simulink model "RCAM_simulation"  (R2021b)
settings: Solver=VariableStepAuto  StartTime=0.0  StopTime=TF  RelTol=1e-3
values from neighbouring files (symbols this model uses):
  h0 = 0    [initializeConstants.m]
  lat0 = convert_coordinates(21, 18, 56.1708)    [initializeConstants.m]
  lon0 = convert_coordinates(157, 51, 29.1348)    [initializeConstants.m]
  u1max = 25*pi/180    (= 0.436332312999)    [initializeConstants.m]
  u1min = -25*pi/180    (= -0.436332312999)    [initializeConstants.m]
  u2max = 10*pi/180    (= 0.174532925199)    [initializeConstants.m]
  u2min = -25*pi/180    (= -0.436332312999)    [initializeConstants.m]
  u3max = 30*pi/180    (= 0.523598775598)    [initializeConstants.m]
  u3min = -30*pi/180    (= -0.523598775598)    [initializeConstants.m]
  u4max = 10*pi/180    (= 0.174532925199)    [initializeConstants.m]
  u4min = 0    [initializeConstants.m]
  u5max = 10*pi/180    (= 0.174532925199)    [initializeConstants.m]
  u5min = 0    [initializeConstants.m]
  udist = [10 ... (first row only)    [initializeConstants.m]
  uo = [0; -0.1780; 0; 0.0821; 0.0821]    [initializeConstants.m]
  x0 = [84.9905; 0; 1.2713; 0; 0; 0; 0; 0.0150; 0]    [initializeConstants.m]
undefined symbols (not defined in the file or in its folder): RCAM_model
libraries: aerolibfltsims x2
settings Model: Creator=khanh  LastModifiedBy=khanh

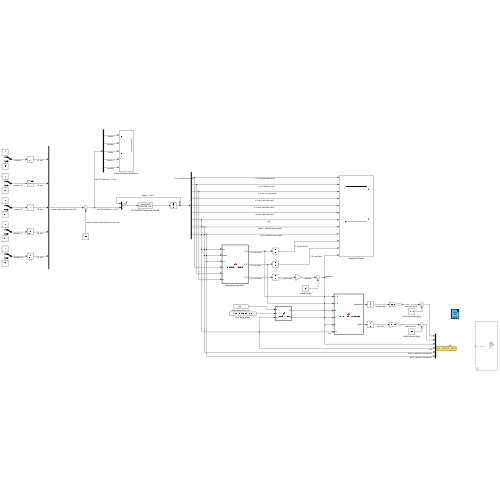
[thumbnail: Simulink's stored preview of the top-level diagram]
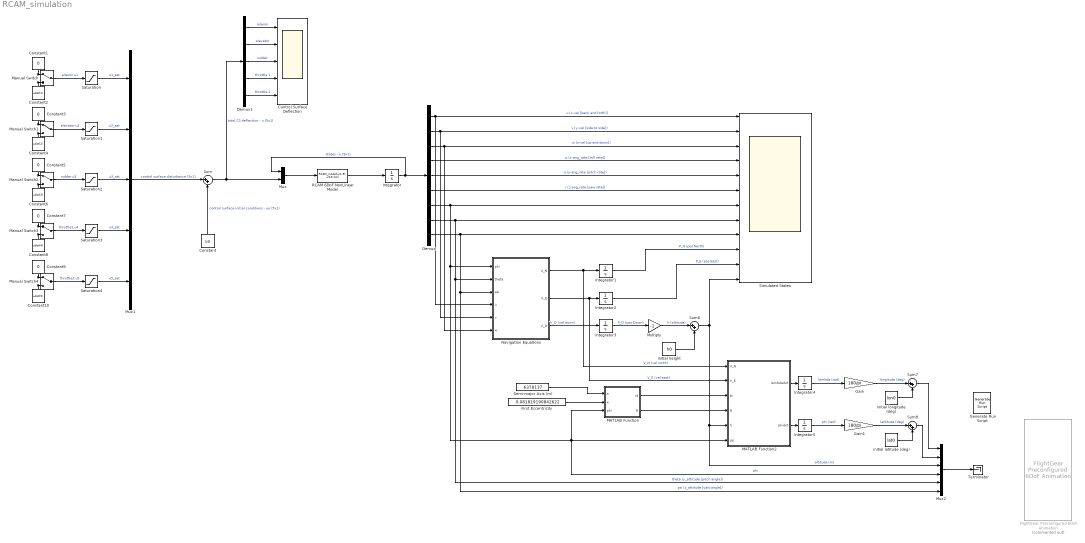
== system RCAM_simulation ==
  Constant : Constant  Value=uo
  Constant{1,3,5,7,9} (5 alike) : Constant  Value=0
  Constant10 : Constant  Value=udist(5)
  Constant2 : Constant  Value=udist(1)
  Constant4 : Constant  Value=udist(2)
  Constant6 : Constant  Value=udist(3)
  Constant8 : Constant  Value=udist(4)
  Control Surface Deflection : Scope  NumInputPorts=5
  Demux : Demux  Outputs=9
  Demux1 : Demux  Outputs=5
  First Eccentricity : Constant  Value=0.081819190842622
  FlightGear Preconfigured 6DoF Animation : aerolibfltsims/FlightGear Preconfigured 6DoF Animation  Commented=on  xFlightGearVersion=v2019.1  DestinationIpAddress=127.0.0.1  DestinationPort=5502  SampleTime=1/30  packetVersion=24
  Gain : Gain  Gain=180/pi
  Gain1 : Gain  Gain=180/pi
  Generate Run Script : aerolibfltsims/Generate Run Script  Architecture=Win64  dataFlow=Send  GeometryModelName=c172p  AirportId=KSFO  RunwayId=10L  InitialAltitude=7224  InitialHeading=113  OffsetDistance=4.72  OffsetAzimuth=0  InstallScenery=off  DisableShaders=on  OriginAddress=127.0.0.1  DestinationPort=5502  OriginPort=5505  LocalAddress=127.0.0.1  OutputFileName=runfg.bat  FlightGearBaseDirectory=C:\Program Files\FlightGear 2020.3
  Integrator : Integrator  InitialCondition=x0
  Integrator{1..4} (4 alike) : Integrator
  Integrator5 : Integrator  UpperSaturationLimit=pi  LowerSaturationLimit=-pi
  MATLAB Function : MATLAB Function  TreatAsAtomicUnit=on
  MATLAB Function2 : MATLAB Function  TreatAsAtomicUnit=on
  Manual Switch{,1..4} (5 alike) : ManualSwitch
  Multiply : Gain  Gain=-1
  Mux : Mux  Inputs=2
  Mux1 : Mux  Inputs=5
  Mux2 : Mux  Inputs=6
  Navigation Equations : MATLAB Function  TreatAsAtomicUnit=on
  RCAM 6DoF NonLinear Model : MATLABFcn  MATLABFcn=RCAM_model(u(1:9), u(10:14))
  Saturation : Saturate  UpperLimit=u1max  LowerLimit=u1min
  Saturation1 : Saturate  UpperLimit=u2max  LowerLimit=u2min
  Saturation2 : Saturate  UpperLimit=u3max  LowerLimit=u3min
  Saturation3 : Saturate  UpperLimit=u4max  LowerLimit=u4min
  Saturation4 : Saturate  UpperLimit=u5max  LowerLimit=u5min
  Semi-major Axis (m) : Constant  Value=6378137
  Simulated States : Scope  NumInputPorts=12
  Sum{,6..8} (4 alike) : Sum  Inputs=|++
  Terminator : Terminator
  initial height : Constant  Value=h0
  initial latitude (deg) : Constant  Value=lat0
  initial longitude (deg) : Constant  Value=lon0
  wires:
  RCAM 6DoF NonLinear Model/1 -> Integrator/1
  Integrator/1 -> Demux/1, Mux/1  "states - x (9x1)"
  Constant/1 -> Sum/2  "control surface initial conditions - uo (5x1)"
  Mux/1 -> RCAM 6DoF NonLinear Model/1
  Sum/1 -> Demux1/1, Mux/2  "total CS deflection - u (5x1)"
  Constant2/1 -> Manual Switch/2
  Constant1/1 -> Manual Switch/1
  Manual Switch/1 -> Saturation/1  "aileron u1"
  Saturation/1 -> Mux1/1  "u1_sat"
  Manual Switch4/1 -> Saturation4/1  "throttle2 u5"
  Saturation4/1 -> Mux1/5  "u5_sat"
  Saturation3/1 -> Mux1/4  "u4_sat"
  Manual Switch3/1 -> Saturation3/1  "throttle1 u4"
  Manual Switch2/1 -> Saturation2/1  "rudder u3"
  Saturation2/1 -> Mux1/3  "u3_sat"
  Saturation1/1 -> Mux1/2  "u2_sat"
  Demux1/1 -> Control Surface Deflection/1  "aileron"
  Demux1/2 -> Control Surface Deflection/2  "elevator"
  Demux1/3 -> Control Surface Deflection/3  "rudder"
  Demux1/4 -> Control Surface Deflection/4  "throttle 1"
  Demux1/5 -> Control Surface Deflection/5  "throttle 2"
  Mux1/1 -> Sum/1  "control surface disturbance (5x1)"
  Demux/1 -> Navigation Equations/4(u), Simulated States/1  "u (x-vel [back and forth])"
  Demux/2 -> Navigation Equations/5(v), Simulated States/2  "v (y-vel [side to side])"
  Demux/3 -> Navigation Equations/6(w), Simulated States/3  "w (z-vel [up and down])"
  Demux/4 -> Simulated States/4  "p (x-ang_rate [roll rate])"
  Demux/5 -> Simulated States/5  "q (y-ang_rate [pitch rate])"
  Demux/6 -> Simulated States/6  "r (z-ang_rate [yaw rate])"
  Demux/8 -> Mux2/5, Navigation Equations/2(theta), Simulated States/8  "theta (y_attitude [pitch angle])"
  Demux/9 -> Mux2/6, Navigation Equations/3(psi), Simulated States/9  "psi (z_attitude [yaw angle])"
  Navigation Equations/3(V_D) -> Integrator3/1  "V_D (vel down)"
  Navigation Equations/2(V_E) -> Integrator2/1, MATLAB Function2/2(V_E)  "V_E (vel east)"
  Navigation Equations/1(V_N) -> MATLAB Function2/1(V_N), Integrator1/1  "V_N (vel north)"
  Integrator1/1 -> Simulated States/10  "P_N (pos North)"
  Integrator2/1 -> Simulated States/11  "P_E (pos East)"
  Integrator3/1 -> Multiply/1  "P_D (pos Down)"
  Semi-major Axis (m)/1 -> MATLAB Function/1(a)
  First Eccentricity/1 -> MATLAB Function/2(e)
  MATLAB Function/2(N) -> MATLAB Function2/4(N)
  MATLAB Function/1(M) -> MATLAB Function2/3(M)
  Demux/7 -> MATLAB Function2/6(psi), MATLAB Function/3(phi), Mux2/4, Navigation Equations/1(phi), Simulated States/7  "phi"
  Integrator5/1 -> Gain1/1  "phi (rad)"
  Integrator4/1 -> Gain/1  "lambda (rad)"
  Gain/1 -> Sum7/1  "longitude (deg)"
  Multiply/1 -> Sum6/1  "h (altitude)"
  Sum6/1 -> Simulated States/12, Mux2/3, MATLAB Function2/5(h)  "altitude (m)"
  initial height/1 -> Sum6/2
  MATLAB Function2/1(lambdadot) -> Integrator4/1
  MATLAB Function2/2(phidot) -> Integrator5/1
  Gain1/1 -> Sum8/1  "lattitude (deg)"
  initial longitude (deg)/1 -> Sum7/2
  initial latitude (deg)/1 -> Sum8/2
  Sum7/1 -> Mux2/1
  Sum8/1 -> Mux2/2
  Constant4/1 -> Manual Switch1/2
  Constant3/1 -> Manual Switch1/1
  Constant6/1 -> Manual Switch2/2
  Constant5/1 -> Manual Switch2/1
  Constant8/1 -> Manual Switch3/2
  Constant7/1 -> Manual Switch3/1
  Constant10/1 -> Manual Switch4/2
  Constant9/1 -> Manual Switch4/1
  Manual Switch1/1 -> Saturation1/1  "elevator u2"
  Mux2/1 -> Terminator/1

== matlab function RCAM_simulation/MATLAB Function ==
  data: a input; M output; e input; phi input; N output
function [M, N] = calculate_mn (a, e, phi)

M = a*(1-e^2)/(1-(e^2)*sin(phi)^2)^1.5;

N = a/(1-(e^2)*sin(phi)^2)^0.5;

end

== matlab function RCAM_simulation/Navigation Equations ==
  data: phi input; theta input; psi input; u input; V_N output; v input; w input; V_E output; V_D output
function [V_N, V_E, V_D] = navigation_equation(phi, theta, psi, u, v, w)

x7 = phi;
x8 = theta;
x9 = psi;
x1 = u;
x2 = v;
x3 = w;

V_b = [x1; x2; x3];

%navigation equations
C1v = [cos(x9) sin(x9) 0; -sin(x9) cos(x9) 0; 0 0 1];

C21 = [cos(x8) 0 -sin(x8); 0 1 0; sin(x8) 0 cos(x8)];

Cb2 = [1 0 0; 0 cos(x7) sin(x7); 0 -sin(x7) cos(x7)];

Cvb = Cb2*C21*C1v;
Cvb = Cvb';

vel_vector = Cvb*V_b;

V_N = vel_vector(1);
V_E = vel_vector(2);
V_D = vel_vector(3);

end

== matlab function RCAM_simulation/MATLAB Function2 ==
  data: lambdadot output; V_N input; V_E input; phidot output; M input; N input; h input; psi input
function [lambdadot, phidot] = calculate_phi_lambdadot(V_N, V_E, M, N, h, psi)

lambdadot = V_E/(N+h)*cos(psi);
phidot = V_N/(M+h);


end
